simulink model "logic_test"  (Simulink 8.4)
settings: Solver=FixedStepDiscrete  StartTime=0.0  StopTime=10.0  FixedStep=1.0  RelTol=1e-3
settings Model: Creator=arnaud  LastModifiedBy=arnaud
settings DataIOCC: SaveFormat=Structure
settings DebuggingCC: StrictBusMsg=Warning

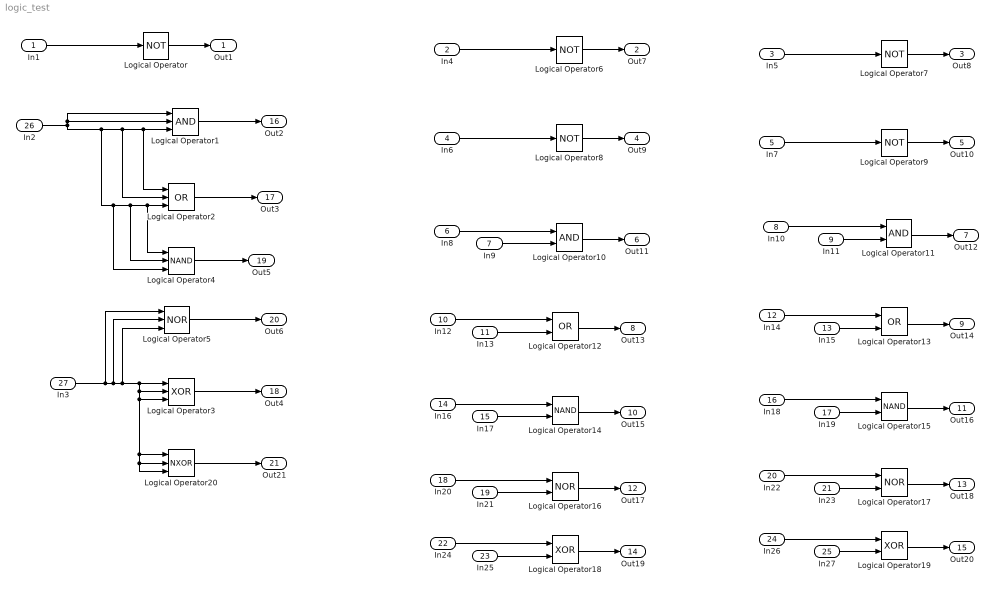
== system logic_test ==
  In1 : Inport
  In4 : Inport  Port=2  OutDataTypeStr=double
  In5 : Inport  Port=3  OutDataTypeStr=int8
  In6 : Inport  Port=4  OutDataTypeStr=double  PortDimensions=2
  In7 : Inport  Port=5  OutDataTypeStr=int8  PortDimensions=[2 3]
  In8 : Inport  Port=6  OutDataTypeStr=double  PortDimensions=2
  In9 : Inport  Port=7  OutDataTypeStr=double  PortDimensions=2
  In10 : Inport  Port=8  OutDataTypeStr=int8  PortDimensions=[2 3]
  In11 : Inport  Port=9  OutDataTypeStr=int8  PortDimensions=[2 3]
  In12 : Inport  Port=10  OutDataTypeStr=double  PortDimensions=2
  In13 : Inport  Port=11  OutDataTypeStr=double  PortDimensions=2
  In14 : Inport  Port=12  OutDataTypeStr=int8  PortDimensions=[2 3]
  In15 : Inport  Port=13  OutDataTypeStr=int8  PortDimensions=[2 3]
  In16 : Inport  Port=14  OutDataTypeStr=double  PortDimensions=2
  In17 : Inport  Port=15  OutDataTypeStr=double  PortDimensions=2
  In18 : Inport  Port=16  OutDataTypeStr=int8  PortDimensions=[2 3]
  In19 : Inport  Port=17  OutDataTypeStr=int8  PortDimensions=[2 3]
  In20 : Inport  Port=18  OutDataTypeStr=double  PortDimensions=2
  In21 : Inport  Port=19  OutDataTypeStr=double  PortDimensions=2
  In22 : Inport  Port=20  OutDataTypeStr=int8  PortDimensions=[2 3]
  In23 : Inport  Port=21  OutDataTypeStr=int8  PortDimensions=[2 3]
  In24 : Inport  Port=22  OutDataTypeStr=double  PortDimensions=2
  In25 : Inport  Port=23  OutDataTypeStr=double  PortDimensions=2
  In26 : Inport  Port=24  OutDataTypeStr=int8  PortDimensions=[2 3]
  In27 : Inport  Port=25  OutDataTypeStr=int8  PortDimensions=[2 3]
  In2 : Inport  Port=26  PortDimensions=[2]
  In3 : Inport  Port=27  PortDimensions=[2 2]
  Logical Operator{,6..9} (5 alike) : Logic  Operator=NOT  AllPortsSameDT=off  OutDataTypeStr=boolean
  Logical Operator1 : Logic  Inputs=3  AllPortsSameDT=off  OutDataTypeStr=boolean
  Logical Operator10 : Logic  AllPortsSameDT=off  OutDataTypeStr=boolean
  Logical Operator11 : Logic  AllPortsSameDT=off  OutDataTypeStr=boolean
  Logical Operator12 : Logic  Operator=OR  AllPortsSameDT=off  OutDataTypeStr=boolean
  Logical Operator13 : Logic  Operator=OR  AllPortsSameDT=off  OutDataTypeStr=boolean
  Logical Operator14 : Logic  Operator=NAND  AllPortsSameDT=off  OutDataTypeStr=boolean
  Logical Operator15 : Logic  Operator=NAND  AllPortsSameDT=off  OutDataTypeStr=boolean
  Logical Operator16 : Logic  Operator=NOR  AllPortsSameDT=off  OutDataTypeStr=boolean
  Logical Operator17 : Logic  Operator=NOR  AllPortsSameDT=off  OutDataTypeStr=boolean
  Logical Operator18 : Logic  Operator=XOR  AllPortsSameDT=off  OutDataTypeStr=boolean
  Logical Operator19 : Logic  Operator=XOR  AllPortsSameDT=off  OutDataTypeStr=boolean
  Logical Operator2 : Logic  Operator=OR  Inputs=3  AllPortsSameDT=off  OutDataTypeStr=boolean
  Logical Operator20 : Logic  Operator=NXOR  Inputs=3  AllPortsSameDT=off  OutDataTypeStr=boolean
  Logical Operator3 : Logic  Operator=XOR  Inputs=3  AllPortsSameDT=off  OutDataTypeStr=boolean
  Logical Operator4 : Logic  Operator=NAND  Inputs=3  AllPortsSameDT=off  OutDataTypeStr=boolean
  Logical Operator5 : Logic  Operator=NOR  Inputs=3  AllPortsSameDT=off  OutDataTypeStr=boolean
  Out1 : Outport
  Out7 : Outport  Port=2
  Out8 : Outport  Port=3
  Out9 : Outport  Port=4
  Out10 : Outport  Port=5
  Out11 : Outport  Port=6
  Out12 : Outport  Port=7
  Out13 : Outport  Port=8
  Out14 : Outport  Port=9
  Out15 : Outport  Port=10
  Out16 : Outport  Port=11
  Out17 : Outport  Port=12
  Out18 : Outport  Port=13
  Out19 : Outport  Port=14
  Out20 : Outport  Port=15
  Out2 : Outport  Port=16
  Out3 : Outport  Port=17
  Out4 : Outport  Port=18
  Out5 : Outport  Port=19
  Out6 : Outport  Port=20
  Out21 : Outport  Port=21
  wires:
  In1/1 -> Logical Operator/1
  Logical Operator/1 -> Out1/1
  In4/1 -> Logical Operator6/1
  Logical Operator6/1 -> Out7/1
  In5/1 -> Logical Operator7/1
  Logical Operator7/1 -> Out8/1
  In6/1 -> Logical Operator8/1
  Logical Operator8/1 -> Out9/1
  In7/1 -> Logical Operator9/1
  Logical Operator9/1 -> Out10/1
  In8/1 -> Logical Operator10/1
  Logical Operator10/1 -> Out11/1
  In9/1 -> Logical Operator10/2
  In10/1 -> Logical Operator11/1
  Logical Operator11/1 -> Out12/1
  In11/1 -> Logical Operator11/2
  In12/1 -> Logical Operator12/1
  Logical Operator12/1 -> Out13/1
  In13/1 -> Logical Operator12/2
  In14/1 -> Logical Operator13/1
  Logical Operator13/1 -> Out14/1
  In15/1 -> Logical Operator13/2
  In16/1 -> Logical Operator14/1
  Logical Operator14/1 -> Out15/1
  In17/1 -> Logical Operator14/2
  In18/1 -> Logical Operator15/1
  Logical Operator15/1 -> Out16/1
  In19/1 -> Logical Operator15/2
  In20/1 -> Logical Operator16/1
  Logical Operator16/1 -> Out17/1
  In21/1 -> Logical Operator16/2
  In22/1 -> Logical Operator17/1
  Logical Operator17/1 -> Out18/1
  In23/1 -> Logical Operator17/2
  In24/1 -> Logical Operator18/1
  Logical Operator18/1 -> Out19/1
  In25/1 -> Logical Operator18/2
  In26/1 -> Logical Operator19/1
  Logical Operator19/1 -> Out20/1
  In27/1 -> Logical Operator19/2
  In2/1 -> Logical Operator1/2, Logical Operator1/1, Logical Operator1/3, Logical Operator2/1, Logical Operator2/2, Logical Operator2/3, Logical Operator4/1, Logical Operator4/2, Logical Operator4/3
  Logical Operator1/1 -> Out2/1
  Logical Operator2/1 -> Out3/1
  Logical Operator3/1 -> Out4/1
  Logical Operator4/1 -> Out5/1
  Logical Operator5/1 -> Out6/1
  In3/1 -> Logical Operator5/1, Logical Operator5/2, Logical Operator3/1, Logical Operator3/2, Logical Operator20/2, Logical Operator20/3, Logical Operator20/1, Logical Operator3/3, Logical Operator5/3
  Logical Operator20/1 -> Out21/1
